simulink model "Glider6"  (R2017b)
settings: Solver=ode4  StartTime=0.0  StopTime=200.0  FixedStep=0.1  RelTol=1e-3
libraries: simulink x1
settings Model: Creator=whsteyn  LastModifiedBy=whsteyn
settings DataIOCC: LimitDataPoints=on  SaveFormat=Array  SignalLoggingSaveFormat=ModelDataLogs
settings OptimizationCC: InitFltsAndDblsToZero=on  LifeSpan=inf
settings DebuggingCC: SaveWithParameterizedLinksMsg=none  UnderspecifiedInitializationDetection=Classic  MergeDetectMultiDrivingBlocksExec=none  SignalResolutionControl=TryResolveAllWithWarning  SolverPrmCheckMsg=warning  MultiTaskDSMMsg=warning  MultiTaskCondExecSysMsg=none  FcnCallInpInsideContextMsg=warning  SFUnexpectedBacktrackingDiag=warning  SFNoUnconditionalDefaultTransitionDiag=warning  SFExecutionAtInitializationDiag=none
settings HardwareCC: ProdBitPerPointer=32  ProdBitPerSizeT=32  ProdBitPerPtrDiffT=32  ProdLargestAtomicFloat=None  ProdIntDivRoundTo=Undefined  ProdEndianess=Unspecified  ProdWordSize=32  ProdHWDeviceType=32-bit Generic
settings ModelReferenceCC: PropagateSignalLabelsOutOfModel=off
settings CodeAppCC: StateflowObjectComments=on
settings GRTTargetCC: TargetFcnLib=ansi_tfl_tmw.mat  TargetLangStandard=C89/C90 (ANSI)  GeneratePreprocessorConditionals=Disable all  CombineOutputUpdateFcns=off  GRTInterface=on
settings ConfigComp: CovMetricSettings=dw  CovHtmlReporting=on  CovSaveCumulativeToWorkspaceVar=on  CovSaveSingleToWorkspaceVar=on  CovExternalEMLEnable=off  CovSFcnEnable=off

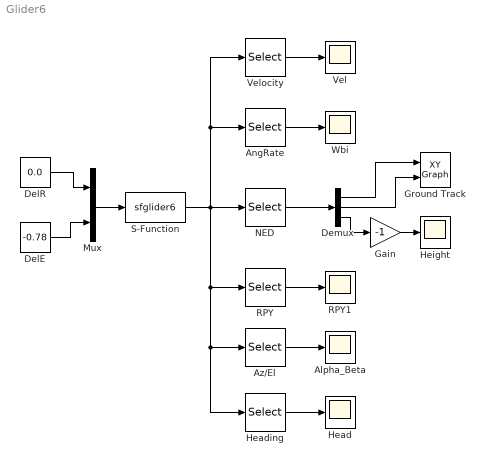
== system Glider6 ==
  Alpha_Beta : Scope
  AngRate : Selector  InputPortWidth=15  IndexOptions=Index vector (dialog)  Indices=[4:6]  OutputSizes=1
  Az/El : Selector  InputPortWidth=15  IndexOptions=Index vector (dialog)  Indices=[13,14]  OutputSizes=1
  DelE : Constant  Value=-0.78
  DelR : Constant  Value=0.0
  Demux : Demux  Outputs=3
  Gain : Gain  Gain=-1
  Ground Track : simulink/Sinks/XY Graph  xmin=-1000  xmax=3000  ymin=-1000  ymax=1000  st=-1
  Head : Scope
  Heading : Selector  InputPortWidth=15  IndexOptions=Index vector (dialog)  Indices=[13,14]  OutputSizes=1
  Height : Scope
  Mux : Mux  Inputs=2
  NED : Selector  InputPortWidth=15  IndexOptions=Index vector (dialog)  Indices=[7:9]  OutputSizes=1
  RPY : Selector  InputPortWidth=15  IndexOptions=Index vector (dialog)  Indices=[10:12]  OutputSizes=1
  RPY1 : Scope
  S-Function : S-Function  FunctionName=sfglider6  Parameters=1000,2.5,[11.25 0 0.8],[0 1.4 0]  SFunctionDeploymentMode=off  EnableBusSupport=off
  Vel : Scope
  Velocity : Selector  InputPortWidth=15  IndexOptions=Index vector (dialog)  Indices=[1:3]  OutputSizes=1
  Wbi : Scope
  wires:
  Mux/1 -> S-Function/1
  S-Function/1 -> AngRate/1, Velocity/1, NED/1, RPY/1, Heading/1, Az/El/1
  NED/1 -> Demux/1
  Velocity/1 -> Vel/1
  DelR/1 -> Mux/1
  Gain/1 -> Height/1
  Demux/3 -> Gain/1
  Demux/1 -> Ground Track/1
  Demux/2 -> Ground Track/2
  Az/El/1 -> Alpha_Beta/1
  AngRate/1 -> Wbi/1
  RPY/1 -> RPY1/1
  DelE/1 -> Mux/2
  Heading/1 -> Head/1
